simulink subsystem "ConvolutionalDecodingLSF"  (R2024b)
settings: Solver=VariableStepAuto  StartTime=0.0  StopTime=10.0  RelTol=1e-3
undefined symbols (not defined in the file or in its folder): Param
libraries: commblkintrlv2 x1, simulink x1, commcnvcod2 x1
settings Model: Creator=fredr  LastModifiedBy=rober

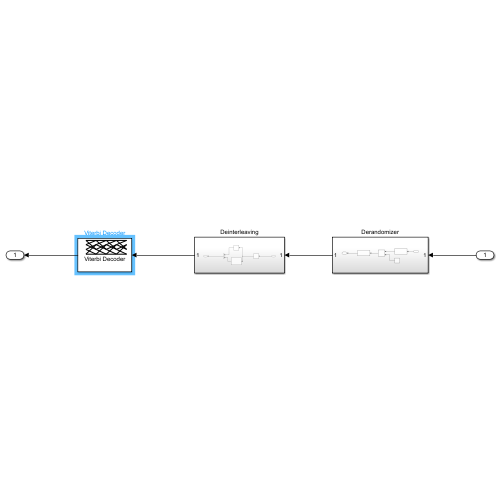
[thumbnail: Simulink's stored preview of the top-level diagram]
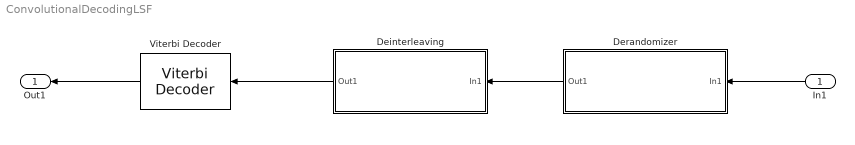
== system ConvolutionalDecodingLSF ==
  In1 : Inport
  Deinterleaving : Subsystem
  Derandomizer : Subsystem
  Viterbi Decoder : commcnvcod2/Viterbi Decoder  trellis=poly2trellis(5, [23 35])  isPunctured=on  punctureVector=Param.Puncturing.P1  erasures=off  dectype=Hard decision  nsdecb=2  runSigValErrCheck=off  tbdepth=20  opmode=Truncated  reset=off  delayedResetAction=on  smWordLength=16  outDataType=double
      settings: LibrarySourceBlock=commhdlcnvcod/Viterbi Decoder
  Out1 : Outport
  wires:
  Derandomizer/1(Out1) -> Deinterleaving/1(In1)
  In1/1 -> Derandomizer/1(In1)
  Viterbi Decoder/1 -> Out1/1
  Deinterleaving/1(Out1) -> Viterbi Decoder/1

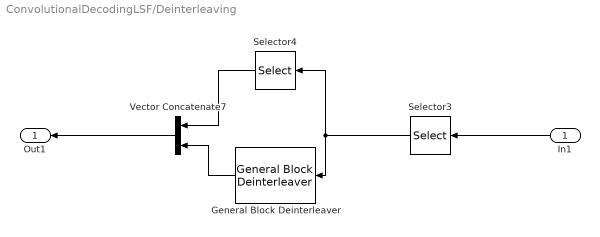
== system ConvolutionalDecodingLSF/Deinterleaving ==
  In1 : Inport
  General Block Deinterleaver : commblkintrlv2/General Block Deinterleaver  StatePerturbationForJacobian=1.0e-05  permutationVectorSource=Dialog  elements=Param.InterleavingTable
  Selector3 : Selector  IndexOptions=Index vector (dialog)  Indices=[2:368]  OutputSizes=1
  Selector4 : Selector  IndexOptions=Index vector (dialog)  Indices=[1]  OutputSizes=1
  Vector Concatenate7 : Concatenate
  Out1 : Outport
  wires:
  Vector Concatenate7/1 -> Out1/1
  In1/1 -> Selector3/1
  General Block Deinterleaver/1 -> Vector Concatenate7/2
  Selector3/1 -> General Block Deinterleaver/1, Selector4/1
  Selector4/1 -> Vector Concatenate7/1

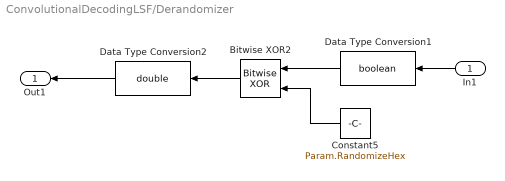
== system ConvolutionalDecodingLSF/Derandomizer ==
  In1 : Inport
  Bitwise XOR2 : simulink/Logic and Bit Operations/Bitwise Operator  logicop=XOR  UseBitMask=off  NumInputPorts=2  BitMask=bin2dec('11011001')  BitMaskRealWorld=Stored Integer
  Constant5 : Constant  Value=Param.RandomizeHex  VectorParams1D=off
  Data Type Conversion1 : DataTypeConversion  OutDataTypeStr=boolean  SaturateOnIntegerOverflow=off  RndMeth=Floor
  Data Type Conversion2 : DataTypeConversion  OutDataTypeStr=double  SaturateOnIntegerOverflow=off  RndMeth=Floor
  Out1 : Outport
  wires:
  In1/1 -> Data Type Conversion1/1
  Data Type Conversion2/1 -> Out1/1
  Bitwise XOR2/1 -> Data Type Conversion2/1
  Data Type Conversion1/1 -> Bitwise XOR2/1
  Constant5/1 -> Bitwise XOR2/2
